simulink model "LLC_model"  (R2026a)
settings: Solver=VariableStepAuto  StopTime=1
libraries: ee_lib x25, fl_lib x23, nesl_utility x6
settings Model: Creator=leone  LastModifiedBy=leone

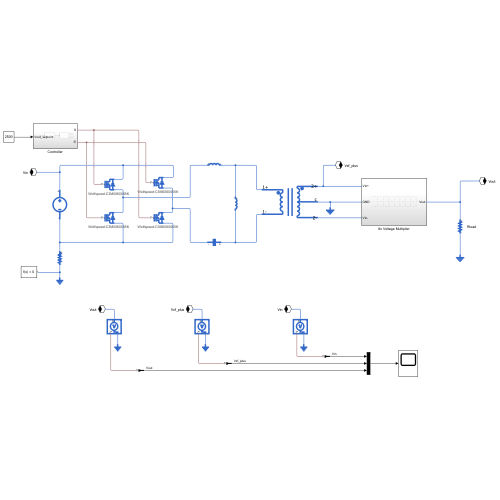
[thumbnail: Simulink's stored preview of the top-level diagram]
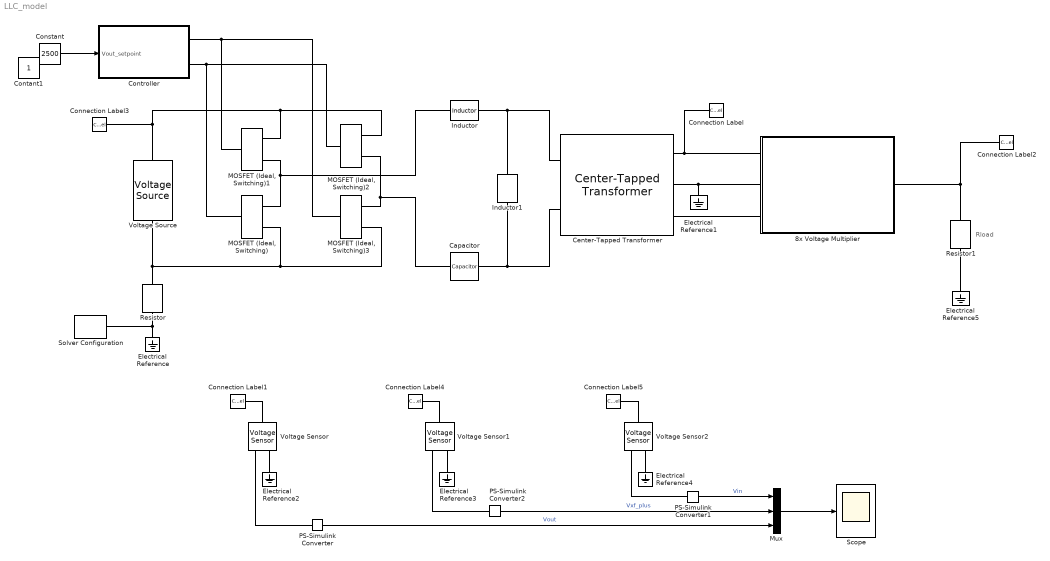
== system LLC_model ==
  note: Rload
  8x Voltage Multiplier : Subsystem
  Capacitor : ee_lib/Passive/Capacitor  cap_option=ee.enum.passive.capacitor.capOption.const  c=250e-9 F  Cvec=[1e-05, 1e-06] F  Vvec=[0, 10] V  CV_table_symmetry=ee.enum.passive.capacitor.tableSymmetry.yes  f_vec=[1, 10] kHz  DFext_vec=[.8, 1.2]  enable_C_tol=ee.enum.toleranceApplication.none  averaging_period=0 s  C_tol=5  tol_distribution=ee.enum.toleranceDistribution.uniform  nSigma=4  r=10 mOhm  g=0 1/Ohm  enable_operating_limits=ee.enum.enable.no  operating_limit_action=ee.enum.passive.reportOpLim.warn  max_working_voltage_range=[-25, 25] V  power_rating=1 W  maxTemperature=85 degC  thermalEnable=false  thermalMass=1 J/K  i_specify=off  i_priority=None  i=0 A  i_nominal_specify=off  i_nominal_value=1  i_nominal_unit=A  v_specify=off  v_priority=None  v=0 V  v_nominal_specify=off  v_nominal_value=1  v_nominal_unit=V  vc_specify=off  vc_priority=High  vc=0 V  vc_nominal_specify=off  vc_nominal_value=1  vc_nominal_unit=V  T_specify=off  T_priority=None  T=298.15 K  T_nominal_specify=off  T_nominal_value=1  T_nominal_unit=K
  Center-Tapped Transformer : ee_lib/Passive/Transformers/Center-Tapped Transformer  modeling_option=ee.enum.transformer_option.ideal  n=1/60  T=0.5  Rw1=0.01 Ohm  L1=0.0001 H  Rw2=0.01 Ohm  L2=0.0001 H  Rm=100 Ohm  Lm=0.04 H  i1_specify=off  i1_priority=None  i1=0 A  i1_nominal_specify=off  i1_nominal_value=1  i1_nominal_unit=A  i2p_specify=off  i2p_priority=None  i2p=0 A  i2p_nominal_specify=off  i2p_nominal_value=1  i2p_nominal_unit=A  i2n_specify=off  i2n_priority=None  i2n=0 A  i2n_nominal_specify=off  i2n_nominal_value=1  i2n_nominal_unit=A
  Connection Label : ConnectionLabel  Label=Vxf_plus
  Connection Label1 : ConnectionLabel  Label=Vout
  Connection Label2 : ConnectionLabel  Label=Vout
  Connection Label3 : ConnectionLabel  Label=Vin
  Connection Label4 : ConnectionLabel  Label=Vxf_plus
  Connection Label5 : ConnectionLabel  Label=Vin
  Constant : Constant  Value=2500
  Controller : Subsystem
  Electrical Reference{,1..5} (6 alike) : fl_lib/Electrical/Electrical Elements/Electrical Reference
  Inductor : ee_lib/Passive/Inductor  l=800e-6 H  enable_L_tol=ee.enum.toleranceApplication.none  L_tol=20  tol_distribution=ee.enum.toleranceDistribution.uniform  nSigma=4  r=0 Ohm  g=1e-9 1/Ohm  enable_operating_limits=ee.enum.enable.no  operating_limit_action=ee.enum.passive.reportOpLim.warn  max_working_current=1 A  power_rating=1 W  i_L_specify=off  i_L_priority=High  i_L=0 A  i_L_nominal_specify=off  i_L_nominal_value=1  i_L_nominal_unit=A
  Inductor1 : ee_lib/Passive/Inductor  l=2.50e-3 H  enable_L_tol=ee.enum.toleranceApplication.none  L_tol=20  tol_distribution=ee.enum.toleranceDistribution.uniform  nSigma=4  r=0 Ohm  g=1e-9 1/Ohm  enable_operating_limits=ee.enum.enable.no  operating_limit_action=ee.enum.passive.reportOpLim.warn  max_working_current=1 A  power_rating=1 W  i_L_specify=off  i_L_priority=High  i_L=0 A  i_L_nominal_specify=off  i_L_nominal_value=1  i_L_nominal_unit=A
  MOSFET (Ideal, Switching){,1..3} (4 alike) : ee_lib/Semiconductors & Converters/MOSFET (Ideal, Switching)  PartSpecification="{\"CollectionId\":\"MW.SimscapeElectrical\",\"CollectionVersion\":\"1.0.0\",\"DatasetId\":\"Wolfspeed|C3M0060065K|simscape.electrical.mosfetIdealSwitching\",\"DisplayName\":\"Wolfspeed:C3M0060065K\"}"  port_option=ee.enum.controlport.ps  Rds=0.06 % Datasheet derived Ohm  Goff=1.53846153846154e-09 % Datasheet derived S  Vth=2.3 % Datasheet derived V  diode_param=ee.enum.semiconductors.protectionDiode.nodynamics  diode_Vf=1.96 % Datasheet derived V  diode_Ron=0.026 % Wolfspeed XML derived Ohm  diode_Goff=1e-05 % Library default S  diode_C=50e-9 % Parameter not set F  diode_iRM=-235 % Parameter not set A  diode_iF=300 % Parameter not set A  diode_idot=-50 % Parameter not set A/us  diode_trr_param=ee.enum.converters.diodeReverseParam.trr_factor  diode_trr_factor=3 % Parameter not set  diode_trr=15 % Parameter not set us  diode_Qrr=1500 % Parameter not set s*uA  ids_specify=off  ids_priority=None  ids=0 A  ids_nominal_specify=off  ids_nominal_value=1  ids_nominal_unit=A  vds_specify=off  vds_priority=None  vds=0 V  vds_nominal_specify=off  vds_nominal_value=1  vds_nominal_unit=V  vgs_specify=off  vgs_priority=None  vgs=0 V  vgs_nominal_specify=off  vgs_nominal_value=1  vgs_nominal_unit=V  thermal_loss_option=ee.enum.converters.thermalLossOption.tabulated2d  Von_data=[-4.94 -3.655 -2.599 -1.45 -0.6361 -0.336 -0.134 0 0.135 0.344 0.712 1.909 4.14 6.838;-6.1394 -4.05915 -2.711 -1.42 -0.594 -0.32 -0.122 0 0.121 0.307 0.626 1.664 3.692 6.273;-7.6271 -6.29626 -4.38 -2.134 -0.857 -0.42 -0.174 0 0.171 0.429 0.868 2.267 5.09 9.299;-8.7716 -7.2407 -5.04 -2.45 -0.987 -0.504 -0.199 0 0.197 0.494 0.998 2.607 5.853 10.693] % Wolfspeed XML derived V  Tj=[-40 25 175 900] % Wolfspeed XML derived degC  Iout_data=[-100 -75 -50 -25 -10 -5 -2 0 2 5 10 25 50 75] % Wolfspeed XML derived A  tabulateWithVds=true  Eon_data=[0 2.4925506e-05 3.0020907e-05 3.5200994e-05 3.9655672e-05 4.4138921e-05 4.8747187e-05 5.3519718e-05 5.8976611e-05;0 2.4164961e-05 2.9236147e-05 3.3749643e-05 3.8301174e-05 4.2764494e-05 4.6698386e-05 5.1602461e-05 5.6753062e-05;0 2.3495333e-05 2.8951831e-05 3.3745437e-05 3.8367892e-05 4.3121152e-05 4.8054902e-05 5.3420573e-05 5.9175378e-05;0 2.3715992e-05 2.9430801e-05 3.4454641e-05 3.9874621e-05 4.5307731e-05 5.065475e-05 5.7771448e-05 6.4903514e-05;0 2.727339e-05 3.3845422e-05 3.9622837e-05 4.5855815e-05 5.2103891e-05 5.8252962e-05 6.6437165e-05 7.4639042e-05] % Wolfspeed XML derived J  Eoff_data=[0 9.67369e-06 1.029884e-05 1.0634933e-05 1.1274169e-05 1.0260412e-05 1.0514001e-05 1.2230396e-05 1.5487576e-05;0 9.842604e-06 9.359904e-06 1.009951e-05 1.0629802e-05 9.604415e-06 9.456493e-06 1.1348542e-05 1.4548e-05;0 8.498942e-06 9.379624e-06 1.0099504e-05 1.0690132e-05 9.552385e-06 9.785154e-06 1.1875369e-05 1.5432185e-05;0 7.557127e-06 9.243456e-06 9.856036e-06 1.0729422e-05 9.523876e-06 9.940175e-06 1.2586824e-05 1.6634352e-05;0 8.690696e-06 1.0629975e-05 1.1334442e-05 1.2338835e-05 1.0952458e-05 1.1431201e-05 1.4474848e-05 1.9129504e-05] % Wolfspeed XML derived J  Eon_data_3D=reshape([0;0;0;0;0;0;0;0;0;0;0;0;0;0;0;0;0;0;0;0;0;0;0;0;0;0;0;0;0;0;0;0;0;0;0;0;0;0;0;0;0;0;0;0;0;0;0;0;0;0;0;0;0;0;0;0;0;0;0;0;0;0;0;0;0;0;0;0;0;0;0;0;0;0;0;0;0;0;0;0;0;0;0;0;0;0;0;0;0;0;0;0;0;0;0;2.4925506e-05;2.4164961e-05;2.3495333e-05;2.3715992e-05;2.727339e-05;3.0020907e-05;2.9236147e-05;2.8951831e-05;2.9430801e-05;3.3845422e-05;3.5200994e-05;3.3749643e-05;3.3745437e-05;3.4454641e-05;3.9622837e-05;3.9655672e-05;3.8301174e-05;3.8367892e-05;3.9874621e-05;4.5855815e-05;4.4138921e-05;4.2764494e-05;4.3121152e-05;4.5307731e-05;5.2103891e-05;4.8747187e-05;4.6698386e-05;4.8054902e-05;5.065475e-05;5.8252962e-05;5.3519718e-05;5.1602461e-05;5.3420573e-05;5.7771448e-05;6.6437165e-05;5.8976611e-05;5.6753062e-05;5.9175378e-05;6.4903514e-05;7.4639042e-05],[5 9 3]) % Wolfspeed XML derived J  Eoff_data_3D=reshape([0;0;0;0;0;0;0;0;0;0;0;0;0;0;0;0;0;0;0;0;0;0;0;0;0;0;0;0;0;0;0;0;0;0;0;0;0;0;0;0;0;0;0;0;0;0;0;0;0;0;0;0;0;0;0;0;0;0;0;0;0;0;0;0;0;0;0;0;0;0;0;0;0;0;0;0;0;0;0;0;0;0;0;0;0;0;0;0;0;0;0;0;0;0;0;9.67369e-06;9.842604e-06;8.498942e-06;7.557127e-06;8.690696e-06;1.029884e-05;9.359904e-06;9.379624e-06;9.243456e-06;1.0629975e-05;1.0634933e-05;1.009951e-05;1.0099504e-05;9.856036e-06;1.1334442e-05;1.1274169e-05;1.0629802e-05;1.0690132e-05;1.0729422e-05;1.2338835e-05;1.0260412e-05;9.604415e-06;9.552385e-06;9.523876e-06;1.0952458e-05;1.0514001e-05;9.456493e-06;9.785154e-06;9.940175e-06;1.1431201e-05;1.2230396e-05;1.1348542e-05;1.1875369e-05;1.2586824e-05;1.4474848e-05;1.5487576e-05;1.4548e-05;1.5432185e-05;1.6634352e-05;1.9129504e-05],[5 9 3]) % Wolfspeed XML derived J  Tj_loss=[25 75 125 175 900] % Wolfspeed XML derived degC  Iout_data_loss=[0 3.62 6.9 10.03 13.25 16.44 19.48 22.52 25.65] % Wolfspeed XML derived A  Vds_loss=[-10 0 400] % Wolfspeed XML derived V  Eon_scalar=22.86e-3 % Parameter not set J  Eoff_scalar=17.14e-3 % Parameter not set J  Voff=300 % Parameter not set V  Iout_scalar=600 % Parameter not set A  useCurrentFromPreviousCycle=true  useVoltageFromPreviousCycle=true  diodeModelType=ee.enum.converters.diodeModelType.tabulated  diodeTableType=ee.enum.diode.tableType.VfMat  diode_ReverseIVType=ee.enum.diode.diodeReverseIV.constant  diode_IfMat=[.07, .12, .19, 1.75, 4.24, 7.32, 11.2; .16, .3, .72, 2.14, 4.02, 6.35, 9.12] % Parameter not set A  diode_VfMat=[0 3.167 5.021 5.741 6.967 8.153 8.989 9.648;0 2.885 4.423 5.092 6.346 7.641 8.575 9.345;0 2.503 3.915 4.544 5.773 7.149 8.197 9.087;0 2.13 3.327 3.862 4.907 6.077 6.968 7.724] % Wolfspeed XML derived V  diode_TjVec=[-40 25 175 900] % Wolfspeed XML derived degC  diode_VfVec=[.5, .7, .9, 1.3, 1.7, 2.1, 2.5] % Parameter not set V  diode_IfVec=[0 0.13 5 10 25 50 75 100] % Wolfspeed XML derived A  diode_IrMat=[1e-06, 2e-06, 5e-06, 1e-05, 2.5e-05, 5e-05, .0001; 2e-06, 5e-06, 1e-05, 4e-05, 8e-05, .0002, .0005] % Parameter not set A  diode_VrMat=[10, 100, 200, 250, 300, 325, 350; 10, 70, 160, 220, 270, 300, 320] % Parameter not set V  diode_VrVec=[10, 20, 40, 50, 70, 80, 100] % Parameter not set V  diode_IrVec=[1e-06, 2e-06, 5e-06, 1e-05, 2e-05, 5e-05, .0001] % Parameter not set A  diode_Vr=-600 % Parameter not set V  diode_Ls=150 % Parameter not set nH  diode_Erec=0.03 % Parameter not set J  diode_rec_loss_model=ee.enum.diode.reverseRecoveryModelTabulateUpTo3D.tabulated2d  diode_ErecVal=0 % Parameter not set J  diode_scaleWithIandV=true  diode_ErecMat=[0 0;0 0] % Wolfspeed XML derived J  diodeErecMat3D=zeros(2, 3, 2) % Parameter not set J  diode_TjrecVec=[25 35] % Wolfspeed XML derived degC  diode_IfrecVec=[0 10] % Wolfspeed XML derived A  diodeVrecVec=[0, 100] % Parameter not set V  diode_IrecVal=10 % Parameter not set A  diode_VrecVal=10 % Wolfspeed XML derived V  diode_tFilter=1 / 1000 / 100 % Parameter not set s  separateThermalPortForDiode=true  thermal_network_parameterization=ee.enum.thermalNetworkTopology.cauer  Rth=[.03, .2] % Parameter not set K/W  Rth_Cauer=[0.181008 0.386142 0.251088 0.202871] % Wolfspeed XML derived K/W  Rth_Foster=[.08, .14, .22, .16] % Parameter not set K/W  thermal_mass_parameterization=ee.enum.thermalNetwork.thermalmass  thermal_mass=[3, 25] % Parameter not set J/K  thermal_mass_Cauer=[0.000689555 0.0034199 0.015973 0.156608] % Wolfspeed XML derived J/K  thermal_mass_Foster=[.001, .005, .05, .5] % Parameter not set J/K  thermal_time_constant=[.1, 5] % Parameter not set s  thermal_time_constant_Cauer=[.1, 1, 5] % Parameter not set s  thermal_time_constant_Foster=[7e-05, .0007, .01, .08] % Parameter not set s  thermal_mass_initial_temperatures=[25, 25] % Parameter not set degC  thermal_mass_initial_temperatures_Cauer=[25 25 25 25] % Wolfspeed XML derived degC  junction_thermal_mass=0.1 % Parameter not set J/K  Tvec_initial_Foster=[25, 25, 25, 25] % Parameter not set degC  RthDiode=[.03, .2] % Parameter not set K/W  RthCauerDiode=[0.181 0.386 0.251 0.2028] % Wolfspeed XML derived K/W  RthFosterDiode=[.03, .2] % Parameter not set K/W  thermalMassDiode=[3, 25] % Parameter not set J/K  thermalMassCauerDiode=[0.00068955 0.0034199 0.01597 0.1566] % Wolfspeed XML derived J/K  thermalMassFosterDiode=[33, 50] % Parameter not set J/K  thermalTauDiode=[.1, 5] % Parameter not set s  thermalTauCauerDiode=[.1, 1, 5] % Parameter not set s  thermalTauFosterDiode=[1, 10] % Parameter not set s  thermalMassInitTempDiode=[25, 25] % Parameter not set degC  thermalMassInitTempCauerDiode=[25 25 25 25] % Wolfspeed XML derived degC  junctionthermalMassDiode=0.1 % Parameter not set J/K  TVecInitialFosterDiode=[25, 25, 25, 25] % Parameter not set degC  no_thermal_network=ee.enum.enable.no  mosfet_junction_temperature_specify=off  mosfet_junction_temperature_priority=None  mosfet_junction_temperature=25 degC  mosfet_junction_temperature_nominal_specify=off  mosfet_junction_temperature_nominal_value=1  mosfet_junction_temperature_nominal_unit=degC  diode_junction_temperature_specify=off  diode_junction_temperature_priority=None  diode_junction_temperature=25 degC  diode_junction_temperature_nominal_specify=off  diode_junction_temperature_nominal_value=1  diode_junction_temperature_nominal_unit=degC  Qj_specify=off  Qj_priority=None  Qj=0 W  Qj_nominal_specify=off  Qj_nominal_value=1  Qj_nominal_unit=W  accumulatedSwitchingLosses_specify=off  accumulatedSwitchingLosses_priority=None  accumulatedSwitchingLosses=0 J
      settings: AttributesFormatString=Wolfspeed:C3M0060065K
  Mux : Mux  Inputs=3
  PS-Simulink Converter : nesl_utility/PS-Simulink Converter  PhysicalDomain=network_engine_domain  SubClassName=ps_output  LeftPortType=input  RightPortType=output  PseudoPeriodic=off  Frequencies=[]  VectorFormat=inherit  Unit=inherit  AffineConversion=off
  PS-Simulink Converter1 : nesl_utility/PS-Simulink Converter  PhysicalDomain=network_engine_domain  SubClassName=ps_output  LeftPortType=input  RightPortType=output  PseudoPeriodic=off  Frequencies=[]  VectorFormat=inherit  Unit=inherit  AffineConversion=off
  PS-Simulink Converter2 : nesl_utility/PS-Simulink Converter  PhysicalDomain=network_engine_domain  SubClassName=ps_output  LeftPortType=input  RightPortType=output  PseudoPeriodic=off  Frequencies=[]  VectorFormat=inherit  Unit=inherit  AffineConversion=off
  Resistor : fl_lib/Electrical/Electrical Elements/Resistor  R=1 GOhm  i_specify=off  i_priority=None  i=0 A  i_nominal_specify=off  i_nominal_value=1  i_nominal_unit=A  v_specify=off  v_priority=None  v=0 V  v_nominal_specify=off  v_nominal_value=1  v_nominal_unit=V
  Resistor1 : fl_lib/Electrical/Electrical Elements/Resistor  R=2.7e6 Ohm  i_specify=off  i_priority=None  i=0 A  i_nominal_specify=off  i_nominal_value=1  i_nominal_unit=A  v_specify=off  v_priority=None  v=0 V  v_nominal_specify=off  v_nominal_value=1  v_nominal_unit=V
  Scope : Scope
      settings: ActiveDisplayYMinimum=1562.5615191032161  ActiveDisplayYMaximum=1569.5441988186874
  Solver Configuration : nesl_utility/Solver Configuration  PhysicalDomain=network_engine_domain  SubClassName=solver  LeftPortType=input  RightPortType=generic  Tones=[]  Harmonics=[]  SimulateNoise=off  Profile=off  UseLocalSampling=off  EnableSwitchedLinearOptims=on  FrequencyDomain=off  UseCCode=off  RelTol=0.001  AbsTol=0.001  MinStep=1e-09  ToWorkspace=off  RevertToSquareIcSolve=off  NumHomotopyIterations=100  PhasorMode=off  PhasorModeNumHarmonics=1  ConsistencySolver=NEWTON_XTOL_AFTER_FTOL  CanonicalOrdering=CANONICAL  OptimizeIntermediates=OPTIMIZED  IndexReductionMethod=DerivativeReplacement  DoDC=off  ResidualTolerance=1e-09  ConsistencyTolSource=GLOBAL  ConsistencyAbsTol=0.001  ConsistencyRelTol=0.001  ConsistencyTolFactor=0.001  UseLocalSolver=off  LocalSolverChoice=NE_BACKWARD_EULER_ADVANCER  ResolveIndetEquations=on  FunctionEvalNumThread=1  LocalSolverSampleTime=0.00000001  DoFixedCost=off  MaxNonlinIter=3  MaxModeIter=2  ComputeImpulses=off  ImpulseIterations=2  LinearAlgebra=auto  LinearAlgebraNumThread=0  EquationFormulation=NE_TIME_EF  DelaysMemoryBudget=1024  AutomaticFiltering=on  FilteringTimeConstant=0.001  PartitionStorageMethod=AS_NEEDED  PartitionMemoryBudget=1024  PartitionMethod=ROBUST  MultibodyUseLocalSolver=off  MultibodyLocalSolverChoice=ODE1  MultibodyLocalSolverSampleTime=0.001
  Voltage Sensor : fl_lib/Electrical/Electrical Sensors/Voltage Sensor
  Voltage Sensor1 : fl_lib/Electrical/Electrical Sensors/Voltage Sensor
  Voltage Sensor2 : fl_lib/Electrical/Electrical Sensors/Voltage Sensor
  Voltage Source : ee_lib/Sources/Voltage Source  dc_voltage=170 V  ac_voltage=0 V  ac_shift=0 rad  ac_frequency=60 Hz  noise_mode=ee.enum.sources.noise.Disabled  PSD=0 V^2/Hz  sample_time=1e-3 s  repeatability=ee.enum.sources.repeatability.NotRepeatable  user_seed=0  auto_seed=3499211588  i_specify=off  i_priority=None  i=0 A  i_nominal_specify=off  i_nominal_value=1  i_nominal_unit=A  v_specify=off  v_priority=None  v=0 V  v_nominal_specify=off  v_nominal_value=1  v_nominal_unit=V
  Contant1 : Constant  IOType=siggen
  wires:
  PS-Simulink Converter/1 -> Mux/3  "Vout"
  PS-Simulink Converter2/1 -> Mux/2  "Vxf_plus"
  PS-Simulink Converter1/1 -> Mux/1  "Vin"
  Mux/1 -> Scope/1
  Constant/1 -> Controller/1(Vout_setpoint)
  connections:
  "MOSFET (Ideal, Switching)1"/RConn2 -- Inductor/LConn1 -- "MOSFET (Ideal, Switching)"/RConn1
  "MOSFET (Ideal, Switching)2"/RConn2 -- "MOSFET (Ideal, Switching)3"/RConn1 -- Capacitor/RConn1
  Voltage Source/LConn1 -- "MOSFET (Ideal, Switching)2"/RConn1 -- "MOSFET (Ideal, Switching)1"/RConn1 -- Connection Label3/LConn1
  "MOSFET (Ideal, Switching)"/RConn2 -- "MOSFET (Ideal, Switching)3"/RConn2 -- Voltage Source/RConn1 -- Resistor/LConn1
  Inductor1/LConn1 -- Center-Tapped Transformer/LConn1 -- Inductor/RConn1
  Inductor1/RConn1 -- Center-Tapped Transformer/LConn2 -- Capacitor/LConn1
  Resistor/RConn1 -- Solver Configuration/RConn1 -- Electrical Reference/LConn1
  Electrical Reference1/LConn1 -- 8x Voltage Multiplier/LConn2 -- Center-Tapped Transformer/RConn2
  8x Voltage Multiplier/LConn1 -- Connection Label/LConn1 -- Center-Tapped Transformer/RConn1
  8x Voltage Multiplier/LConn3 -- Center-Tapped Transformer/RConn3
  8x Voltage Multiplier/RConn1 -- Connection Label2/LConn1 -- Resistor1/LConn1
  PS-Simulink Converter/LConn1 -- Voltage Sensor/RConn1
  Electrical Reference2/LConn1 -- Voltage Sensor/RConn2
  Voltage Sensor/LConn1 -- Connection Label1/LConn1
  PS-Simulink Converter2/LConn1 -- Voltage Sensor1/RConn1
  Voltage Sensor1/LConn1 -- Connection Label4/LConn1
  Electrical Reference3/LConn1 -- Voltage Sensor1/RConn2
  Electrical Reference4/LConn1 -- Voltage Sensor2/RConn2
  PS-Simulink Converter1/LConn1 -- Voltage Sensor2/RConn1
  Voltage Sensor2/LConn1 -- Connection Label5/LConn1
  Electrical Reference5/LConn1 -- Resistor1/RConn1
  Controller/RConn1 -- "MOSFET (Ideal, Switching)1"/LConn1 -- "MOSFET (Ideal, Switching)3"/LConn1
  Controller/RConn2 -- "MOSFET (Ideal, Switching)"/LConn1 -- "MOSFET (Ideal, Switching)2"/LConn1

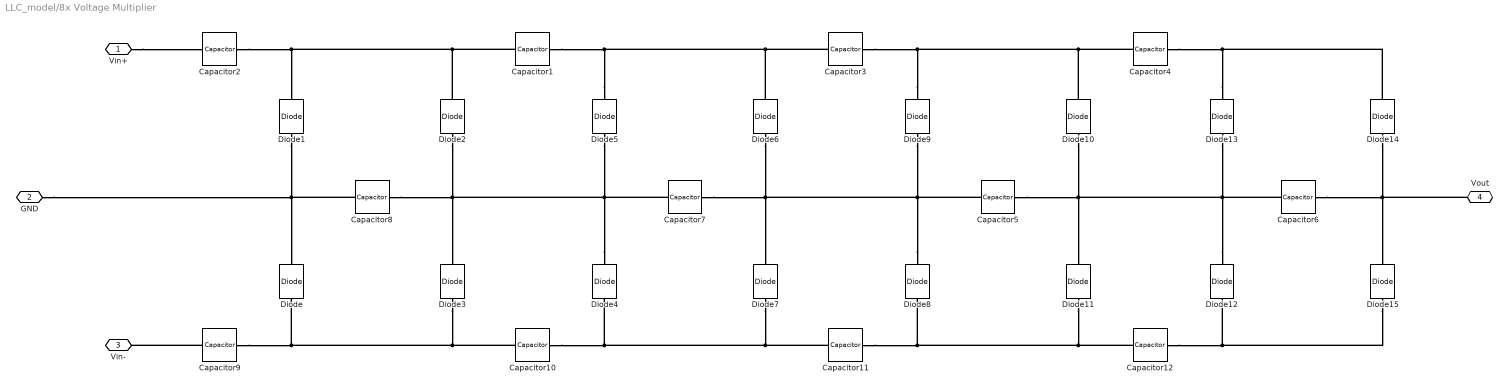
== system LLC_model/8x Voltage Multiplier ==
  Capacitor{1..12} (12 alike) : fl_lib/Electrical/Electrical Elements/Capacitor  c=100e-9 F  r=1e-6 Ohm  g=0 1/Ohm  i_specify=off  i_priority=None  i=0 A  i_nominal_specify=off  i_nominal_value=1  i_nominal_unit=A  v_specify=off  v_priority=None  v=0 V  v_nominal_specify=off  v_nominal_value=1  v_nominal_unit=V  vc_specify=off  vc_priority=High  vc=0 V  vc_nominal_specify=off  vc_nominal_value=1  vc_nominal_unit=V
  Diode{,1..15} (16 alike) : ee_lib/Semiconductors & Converters/Diode  ModelType=ee.enum.diode.modelType.pwl  TableType=ee.enum.diode.tableType.IfMat  IfMat=[.07, .12, .19, 1.75, 4.24, 7.32, 11.2; .16, .3, .72, 2.14, 5.02, 8.35, 13.12] A  VfMat=[.9, 1.15, 1.25, 1.5, 1.75, 2.17, 2.6, 2.85; .58, .68, .75, 1.1, 1.38, 1.77, 2.27, 2.7] V  TjVec=[25, 125] degC  VfVec=[.5, .7, .9, 1.3, 1.7, 2.1, 2.5] V  IfVec=[.1, .2, .5, 1, 2, 4, 7, 10] A  IrMat=[1e-06, 2e-06, 5e-06, 1e-05, 2.5e-05, 5e-05, .0001; 2e-06, 5e-06, 1e-05, 4e-05, 8e-05, .0002, .0005] A  VrMat=[10, 100, 200, 250, 300, 325, 350; 10, 70, 160, 220, 270, 300, 320] V  VrVec=[10, 20, 40, 50, 70, 80, 100] V  IrVec=[1e-06, 2e-06, 5e-06, 1e-05, 2e-05, 5e-05, .0001] A  Vf=0.6 V  Ron=0.3 Ohm  Goff=1e-8 S  prmExp=ee.enum.diode.expParam.useTwo  I12=[.0137, .545] A  V12=[.6, .7] V  RS=0 Ohm  Tmeas=298.15 K  IS=1e-12 A  ec=1  I1=0.0137 A  V1=0.6 V  N_series=1  N_parallel=1  ZenerEnable=false  Rz=0.3 Ohm  BV=30 V  C_param=ee.enum.diode.capParam.fixed  CJ=0 pF  CJ0=5 pF  Vvec=[.1, 10, 100] V  Cvec=[3.5, 1, .4] pF  VJ=1 V  Mgrad=0.5  FC=0.5  Q_param=ee.enum.diode.recoveryParam.off  iRM=-7.15 A  iF=4 A  didt=-750 A/us  trr_factor=3  trr=115 ns  Qrr=150 nA*s  Vr=-600 V  Ls=150 nH  Erec=0.03 J  TT=50 ns  tau=100 ns  T_param=ee.enum.diode.temperatureParam.off  Tdevice=298.15 K  I1_T2=0.245 A  V1_T2=0.5 V  IS_T2=1.25e-7 A  Tmeas2=125 degC  XTI_param=ee.enum.diode.xtiParam.pn  XTI=3  EG_param=ee.enum.diode.egapParam.material_si  EG=1.11 eV  dBVdT=0 V/K  enable_fault_input=simscape.enum.onoff.off  i_specify=off  i_priority=None  i=0 A  i_nominal_specify=off  i_nominal_value=1  i_nominal_unit=A  v_specify=off  v_priority=None  v=0 V  v_nominal_specify=off  v_nominal_value=1  v_nominal_unit=V  v_capacitor_specify=off  v_capacitor_priority=None  v_capacitor=0 V  v_capacitor_nominal_specify=off  v_capacitor_nominal_value=1  v_capacitor_nominal_unit=V  Qj_specify=off  Qj_priority=High  Qj=0 C  Qj_nominal_specify=off  Qj_nominal_value=1  Qj_nominal_unit=C  i_diode_specify=off  i_diode_priority=None  i_diode=0 A  i_diode_nominal_specify=off  i_diode_nominal_value=1  i_diode_nominal_unit=A  v_diode_specify=off  v_diode_priority=None  v_diode=0 V  v_diode_nominal_specify=off  v_diode_nominal_value=1  v_diode_nominal_unit=V  i_capacitor_specify=off  i_capacitor_priority=None  i_capacitor=0 A  i_capacitor_nominal_specify=off  i_capacitor_nominal_value=1  i_capacitor_nominal_unit=A  fidelity_level=ee.enum.diode.fidelity.includeChargeDyn  rec_loss_model=ee.enum.diode.reverseRecoveryModelTabulateUpTo3D.fixed  ErecVal=0 J  scaleWithIandV=true  ErecMat=zeros(2, 3) J  ErecMat3D=zeros(2, 3, 2) J  TjrecVec=[298.15, 398.15] K  IfrecVec=[.1, 1, 10] A  IrecVal=10 A  VrecVal=10 V  VrecVec=[0, 100] V  tFilter=1 / 1000 / 100 s  thermal_network_parameterization=ee.enum.thermalNetworkTopology.junctionCase  Rth=[0, 10] K/W  Rth_Cauer=[1, 3, 10] K/W  Rth_Foster=[.08, .14, .22, .16] K/W  thermal_mass_parameterization=ee.enum.thermalNetwork.timeconstant  thermal_mass=[0, 1] J/K  thermal_mass_Cauer=[.1, .3, 1] J/K  thermal_mass_Foster=[.001, .005, .05, .5] J/K  thermal_time_constant=[0, 10] s  thermal_time_constant_Cauer=[1, 3, 10] s  thermal_time_constant_Foster=[7e-05, .0007, .01, .08] s  thermal_mass_initial_temperatures=[25, 25] degC  thermal_mass_initial_temperatures_Cauer=[25, 25, 25] degC  junction_thermal_mass=0.01 J/K  Tvec_initial_Foster=[25, 25, 25, 25] degC  no_thermal_network=0  junction_temperature_specify=off  junction_temperature_priority=None  junction_temperature=25 degC  junction_temperature_nominal_specify=off  junction_temperature_nominal_value=1  junction_temperature_nominal_unit=degC
  Vin+ : PMIOPort  Side=Left
  GND : PMIOPort  Port=2  Side=Left
  Vin- : PMIOPort  Port=3  Side=Left
  Vout : PMIOPort  Port=4  Side=Right
  connections:
  Diode1/RConn1 -- Capacitor8/LConn1 -- GND/RConn1 -- Diode/RConn1
  Diode/LConn1 -- Capacitor9/RConn1 -- Capacitor10/LConn1 -- Diode3/LConn1
  Vin+/RConn1 -- Capacitor2/LConn1
  Capacitor2/RConn1 -- Capacitor1/LConn1 -- Diode2/RConn1 -- Diode1/LConn1
  Capacitor9/LConn1 -- Vin-/RConn1
  Diode4/RConn1 -- Capacitor7/LConn1 -- Capacitor8/RConn1 -- Diode3/RConn1 -- Diode2/LConn1 -- Diode5/RConn1
  Diode8/RConn1 -- Capacitor5/LConn1 -- Capacitor7/RConn1 -- Diode7/RConn1 -- Diode6/LConn1 -- Diode9/RConn1
  Diode5/LConn1 -- Capacitor1/RConn1 -- Capacitor3/LConn1 -- Diode6/RConn1
  Diode4/LConn1 -- Capacitor10/RConn1 -- Capacitor11/LConn1 -- Diode7/LConn1
  Diode12/RConn1 -- Capacitor6/LConn1 -- Capacitor5/RConn1 -- Diode11/RConn1 -- Diode10/LConn1 -- Diode13/RConn1
  Diode14/LConn1 -- Capacitor6/RConn1 -- Diode15/RConn1 -- Vout/RConn1
  Diode13/LConn1 -- Capacitor4/RConn1 -- Diode14/RConn1
  Diode12/LConn1 -- Capacitor12/RConn1 -- Diode15/LConn1
  Diode8/LConn1 -- Capacitor11/RConn1 -- Capacitor12/LConn1 -- Diode11/LConn1
  Diode9/LConn1 -- Capacitor3/RConn1 -- Capacitor4/LConn1 -- Diode10/RConn1

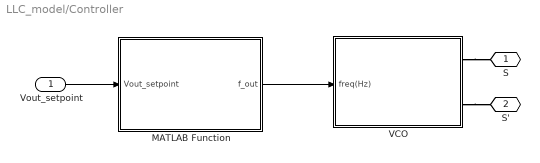
== system LLC_model/Controller ==
  Vout_setpoint : Inport
  MATLAB Function : MATLAB Function  TreatAsAtomicUnit=on
  VCO : Subsystem
  S : PMIOPort  Side=Right
  S' : PMIOPort  Port=2  Side=Right
  wires:
  MATLAB Function/1(f_out) -> VCO/1(freq(Hz))
  Vout_setpoint/1 -> MATLAB Function/1(Vout_setpoint)
  connections:
  VCO/RConn1 -- S/RConn1
  VCO/RConn2 -- S'/RConn1

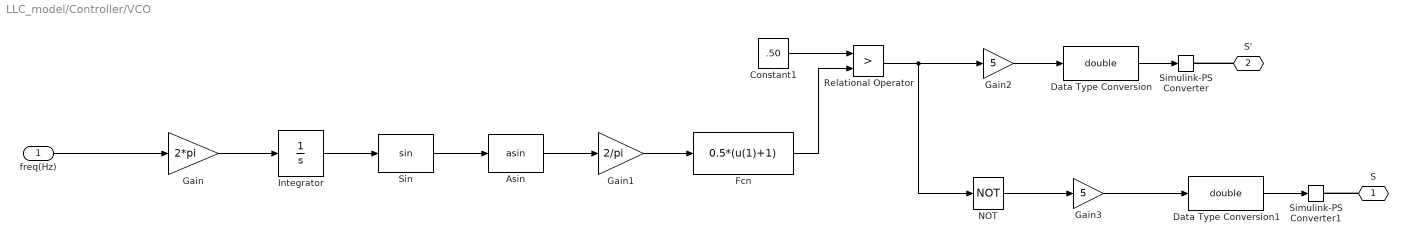
== system LLC_model/Controller/VCO ==
  freq(Hz) : Inport
  Asin : Trigonometry  Operator=asin
  Constant1 : Constant  Value=.50
  Data Type Conversion : DataTypeConversion  OutDataTypeStr=double  SaturateOnIntegerOverflow=off  RndMeth=Floor
  Data Type Conversion1 : DataTypeConversion  OutDataTypeStr=double  SaturateOnIntegerOverflow=off  RndMeth=Floor
  Fcn : Fcn  Expr=0.5*(u(1)+1)
  Gain : Gain  Gain=2*pi
  Gain1 : Gain  Gain=2/pi
  Gain2 : Gain  Gain=5
  Gain3 : Gain  Gain=5
  Integrator : Integrator
  NOT : Logic  Operator=NOT  IconShape=distinctive  AllPortsSameDT=off  OutDataTypeStr=boolean
  Relational Operator : RelationalOperator  Operator=>  OutDataTypeStr=boolean  RndMeth=Simplest  InputSameDT=off
  Simulink-PS Converter : nesl_utility/Simulink-PS Converter  PhysicalDomain=network_engine_domain  SubClassName=ps_input  LeftPortType=input  RightPortType=output  PseudoPeriodic=off  Frequencies=[]  NoiseDistribution=none  NoiseParameters=[]  Unit=1  AffineConversion=off  FilteringAndDerivatives=provide  SimscapeFilterOrder=1  InputFilterTimeConstant=0.001  UdotUserProvided=0
  Simulink-PS Converter1 : nesl_utility/Simulink-PS Converter  PhysicalDomain=network_engine_domain  SubClassName=ps_input  LeftPortType=input  RightPortType=output  PseudoPeriodic=off  Frequencies=[]  NoiseDistribution=none  NoiseParameters=[]  Unit=1  AffineConversion=off  FilteringAndDerivatives=provide  SimscapeFilterOrder=1  InputFilterTimeConstant=0.001  UdotUserProvided=0
  Sin : Trigonometry
  S : PMIOPort  Side=Right
  S' : PMIOPort  Port=2  Side=Right
  wires:
  NOT/1 -> Gain3/1
  Relational Operator/1 -> NOT/1, Gain2/1
  Integrator/1 -> Sin/1
  Gain1/1 -> Fcn/1
  Gain2/1 -> Data Type Conversion/1
  Data Type Conversion/1 -> Simulink-PS Converter/1
  freq(Hz)/1 -> Gain/1
  Data Type Conversion1/1 -> Simulink-PS Converter1/1
  Gain3/1 -> Data Type Conversion1/1
  Asin/1 -> Gain1/1
  Constant1/1 -> Relational Operator/1
  Sin/1 -> Asin/1
  Fcn/1 -> Relational Operator/2
  Gain/1 -> Integrator/1
  connections:
  S'/RConn1 -- Simulink-PS Converter/RConn1
  S/RConn1 -- Simulink-PS Converter1/RConn1

== matlab function LLC_model/Controller/MATLAB Function ==
  data: Vout_setpoint input; f_out output
function f_out = llc_freq_for_vout(Vout_setpoint) %#codegen
%LLC_FREQ_FOR_VOUT  Switching frequency needed for a target output voltage.
%
%   f_out = LLC_FREQ_FOR_VOUT(Vout_setpoint) returns the frequency [Hz] at
%   which the resonant tank's FHA steady-state output amplitude |v_R1|
%   equals Vout_setpoint [V], bounded to [10 kHz, 80 kHz].
%
%   Setpoint convention: PEAK amplitude of the fundamental output voltage.
%   For an RMS target, pass Vout_setpoint_rms*sqrt(2).
%
%   Written for use inside a Simulink MATLAB Function block: fully
%   fixed-size, no fzero / arrayfun / variable-size arrays, so it is
%   MATLAB Coder compatible. Vout_setpoint must be a scalar double.

    % ---- Tank / source constants (from the reference script) -----------
    Ll = 800e-6;  C = 250e-9;  Lm = 2.63e-3;
    N  = 1/30;    R = 50e3;    Vg = 170;

    % ---- Scale setpoint to voltage multiplier output -------------------
    %Vout_setpoint = Vout_setpoint/8;

    % ---- Derived quantities -------------------------------------------
    Re  = (8/pi^2)*R;          % effective ac load (secondary side)
    Rac = N^2*Re;              % load reflected to primary
    Vin = 4*Vg/pi;             % FHA tank-drive amplitude [V]

    % ---- State-space model (fixed size) -------------------------------
    A = [ -Rac/Ll , -1/Ll ,  Rac/Ll ;
           1/C    ,  0    ,  0      ;
           Rac/Lm ,  0    , -Rac/Lm ];
    B    = [ 1/Ll ; 0 ; 0 ];
    Cmat = [ N*Re , 0 , -N*Re ];

    % ---- Frequency band and fixed-size scan grid ----------------------
    f_lo = 10e3;  f_hi = 80e3;
    Ng   = 400;                          % fixed number of grid points
    fg   = linspace(f_lo, f_hi, Ng);     % fixed-size row vector
    vg   = zeros(1, Ng);
    for i = 1:Ng
        vg(i) = vout_at(fg(i), A, B, Cmat, Vin);
    end

    % ---- Locate the gain peak (~series resonance) ---------------------
    ipk = 1;
    for i = 2:Ng
        if vg(i) > vg(ipk)
            ipk = i;
        end
    end

    % ---- Prefer the above-resonance (falling) branch ------------------
    [found, fa, fb] = first_bracket(fg, vg, Vout_setpoint, ipk, Ng);
    if ~found
        % Fall back to a full-band search
        [found, fa, fb] = first_bracket(fg, vg, Vout_setpoint, 1, Ng);
    end

    if found
        % ---- Fixed-count bisection refinement -------------------------
        va = vout_at(fa, A, B, Cmat, Vin) - Vout_setpoint;
        for it = 1:40
            fm = 0.5*(fa + fb);
            vm = vout_at(fm, A, B, Cmat, Vin) - Vout_setpoint;
            if sign(vm) == sign(va)
                fa = fm;  va = vm;
            else
                fb = fm;
            end
        end
        f_out = 0.5*(fa + fb);
    else
        % ---- Unreachable setpoint: clamp to closest grid point --------
        best = 1;
        for i = 2:Ng
            if abs(vg(i) - Vout_setpoint) < abs(vg(best) - Vout_setpoint)
                best = i;
            end
        end
        f_out = fg(best);
    end

    % ---- Enforce bounds ------------------------------------------------
    if f_out < f_lo, f_out = f_lo; end
    if f_out > f_hi, f_out = f_hi; end
end

% ------------------------------------------------------------------------
function v = vout_at(f, A, B, Cmat, Vin)
%VOUT_AT  Steady-state output amplitude at frequency f [Hz].
    M = (1j*2*pi*f)*eye(3) - A;      % complex 3x3, fixed size
    H = Cmat*(M\B);                  % complex scalar
    v = abs(H)*Vin;                  % real amplitude [V]
end

% ------------------------------------------------------------------------
function [found, fa, fb] = first_bracket(fg, vg, target, i0, Ng)
%FIRST_BRACKET  First adjacent grid pair straddling the setpoint from i0 up.
    found = false;
    fa = fg(1);  fb = fg(1);
    prev = sign(vg(i0) - target);
    for i = i0+1:Ng
        cur = sign(vg(i) - target);
        if cur ~= prev && prev ~= 0
            found = true;
            fa = fg(i-1);
            fb = fg(i);
            return;
        end
        prev = cur;
    end
end
